simulink model "Semana_2_Automatizacion_III_2"  (R2025a)
settings: Solver=VariableStepAuto  StartTime=0.0  StopTime=10.0  RelTol=1e-3
settings Model: Creator=jupa_  LastModifiedBy=jupa_

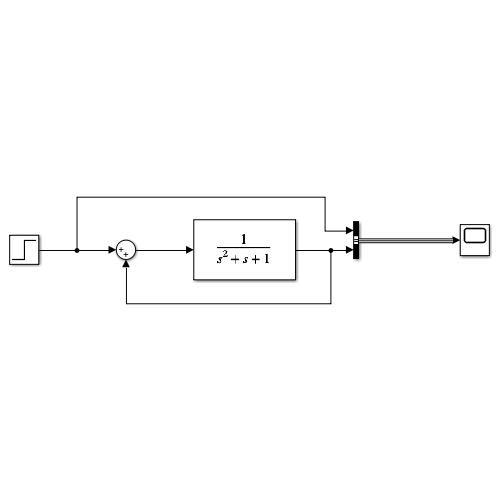
[thumbnail: Simulink's stored preview of the top-level diagram]
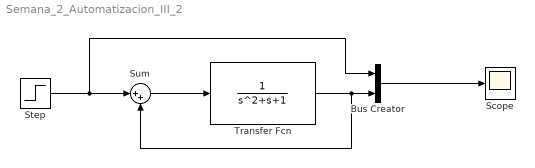
== system Semana_2_Automatizacion_III_2 ==
  Bus Creator : BusCreator  Inputs=2
  Scope : Scope
      settings: ActiveDisplayYMinimum=-1.0000154262426846  ActiveDisplayYMaximum=9.0001388361841634
  Step : Step  SampleTime=0
  Sum : Sum  Inputs=|++
  Transfer Fcn : TransferFcn  Denominator=[1 1 1]
  wires:
  Transfer Fcn/1 -> Sum/2, Bus Creator/2
  Bus Creator/1 -> Scope/1
  Step/1 -> Bus Creator/1, Sum/1
  Sum/1 -> Transfer Fcn/1
